simulink model "task1"  (R2015a)
settings: Solver=ode45  StartTime=0.0  StopTime=10.0  RelTol=1e-3
settings Model: Creator=MANSOOR  LastModifiedBy=Amir

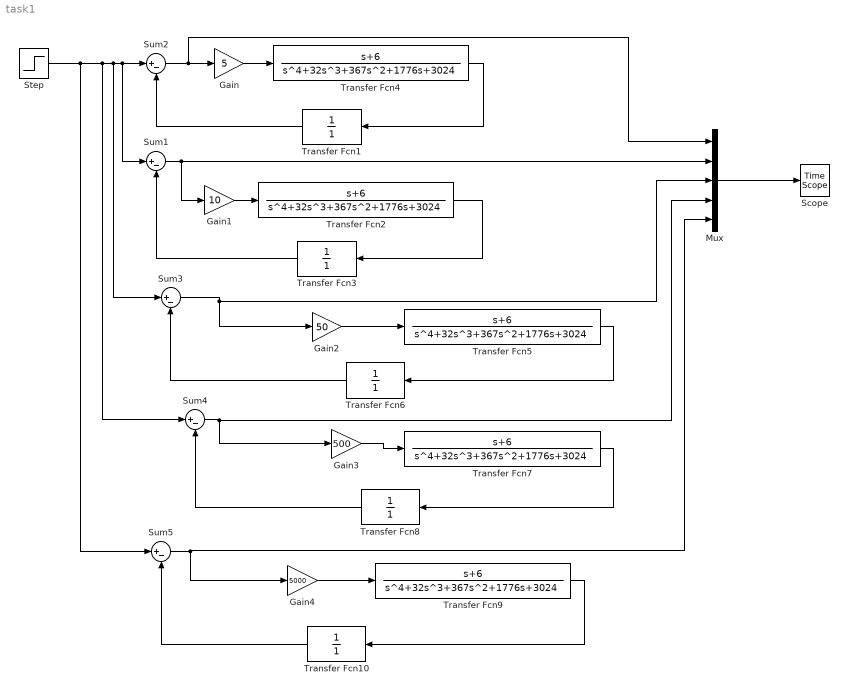
== system task1 ==
  Gain : Gain  Gain=5
  Gain1 : Gain  Gain=10
  Gain2 : Gain  Gain=50
  Gain3 : Gain  Gain=500
  Gain4 : Gain  Gain=5000
  Mux : Mux  Inputs=5
  Scope : TimeScope
  Step : Step  After=5  SampleTime=0
  Sum{1..5} (5 alike) : Sum  Inputs=|+-
  Transfer Fcn{1,3,6,8,10} (5 alike) : TransferFcn  Denominator=[1]
  Transfer Fcn{2,4..5,7,9} (5 alike) : TransferFcn  Numerator=[1 6]  Denominator=[1 32 367 1776 3024]
  wires:
  Gain/1 -> Transfer Fcn4/1
  Sum2/1 -> Mux/1, Gain/1
  Transfer Fcn4/1 -> Transfer Fcn1/1
  Transfer Fcn1/1 -> Sum2/2
  Transfer Fcn2/1 -> Transfer Fcn3/1
  Gain1/1 -> Transfer Fcn2/1
  Sum1/1 -> Gain1/1, Mux/2
  Transfer Fcn3/1 -> Sum1/2
  Mux/1 -> Scope/1
  Transfer Fcn5/1 -> Transfer Fcn6/1
  Gain2/1 -> Transfer Fcn5/1
  Sum3/1 -> Gain2/1, Mux/3
  Transfer Fcn6/1 -> Sum3/2
  Transfer Fcn7/1 -> Transfer Fcn8/1
  Gain3/1 -> Transfer Fcn7/1
  Sum4/1 -> Gain3/1, Mux/4
  Transfer Fcn8/1 -> Sum4/2
  Transfer Fcn9/1 -> Transfer Fcn10/1
  Gain4/1 -> Transfer Fcn9/1
  Sum5/1 -> Gain4/1, Mux/5
  Transfer Fcn10/1 -> Sum5/2
  Step/1 -> Sum5/1, Sum4/1, Sum3/1, Sum1/1, Sum2/1
